simulink model "Discrete_Time_Integrator_verif"  (Simulink 7.2)
settings: Solver=ode45  StartTime=0.0  StopTime=10.0  RelTol=1e-3
settings Model: Creator=Romain  LastModifiedBy=Romain
settings OptimizationCC: ExpressionDepthLimit=128
settings DebuggingCC: SolverPrmCheckMsg=none  FcnCallInpInsideContextMsg=Enable All  StateNameClashWarn=none  StrictBusMsg=ErrorLevel1
settings CodeAppCC: CustomSymbolStrType=$N$R$M_T
settings GRTTargetCC: TargetFunctionLibrary=C89/C90 (ANSI)

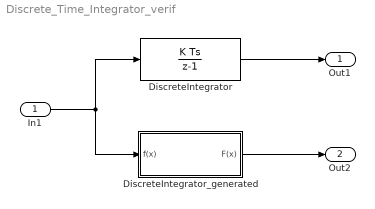
== system Discrete_Time_Integrator_verif ==
  In1 : Inport  OutDataTypeStr=double  DataType=double
  DiscreteIntegrator : DiscreteIntegrator  InitialConditionMode=State only (most efficient)
  DiscreteIntegrator_generated : Subsystem  TreatAsAtomicUnit=on
  Out1 : Outport
  Out2 : Outport  Port=2
  wires:
  In1/1 -> DiscreteIntegrator_generated/1(f(x)), DiscreteIntegrator/1
  DiscreteIntegrator/1 -> Out1/1
  DiscreteIntegrator_generated/1(F(x)) -> Out2/1

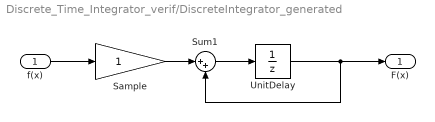
== system Discrete_Time_Integrator_verif/DiscreteIntegrator_generated ==
  f(x) : Inport
  Sample : Gain
  Sum1 : Sum  RequirementInfo={} %GIDa_2dee348c_5ff0_4fe0_aac7_1f1b830464f9  Inputs=|++
  UnitDelay : UnitDelay
  F(x) : Outport  RequirementInfo={} %GIDa_965eaeea_be94_4f12_af28_212c07f723da
  wires:
  f(x)/1 -> Sample/1
  UnitDelay/1 -> Sum1/2, F(x)/1
  Sum1/1 -> UnitDelay/1
  Sample/1 -> Sum1/1
